simulink model "quadFly"  (R2019b)
settings: Solver=ode4  StartTime=0.0  StopTime=inf  FixedStep=0.001  RelTol=1e-3
InitFcn:
  | Init_control;
values from neighbouring files (symbols this model uses):
  Kd_RP_AgngleRate = 0.005    [Init_control.m]    (also in quadFly.sldd)
  Kd_YAW_AngleRate = 0.05    [Init_control.m]    (also in quadFly.sldd)
  Ki_RP_AgngleRate = 0.01    [Init_control.m]    (also in quadFly.sldd)
  Ki_YAW_AngleRate = 0.8    [Init_control.m]    (also in quadFly.sldd)
  Kp_RP_AgngleRate = 0.55    [Init_control.m]    (also in quadFly.sldd)
  Kp_RP_ANGLE = 6.5    [Init_control.m]    (also in quadFly.sldd)
  Kp_YAW_AngleRate = 3.2    [Init_control.m]    (also in quadFly.sldd)
  MAX_CONTROL_ANGLE_RATE_Y = 90    [Init_control.m]    (also in quadFly.sldd = 90.0)
  ModelInit_RPM = 0.0    [quadFly.sldd]
  ModelParam_envAltitude = -41.5260009765625    [quadFly.sldd]
  ModelParam_GlobalNoiseGainSwitch = 1.0    [quadFly.sldd]
  ModelParam_GPSLatLong = 40.1540302 116.2593683    [quadFly.sldd]
  ModelParam_motorCr = 1148.0    [quadFly.sldd]
  ModelParam_motorJm = 0.0001287    [quadFly.sldd]
  ModelParam_motorMinThr = 0.05    [quadFly.sldd]
  ModelParam_motorT = 0.02    [quadFly.sldd]
  ModelParam_motorWb = -141.4    [quadFly.sldd]
  ModelParam_rotorCm = 1.779E-7    [quadFly.sldd]
  ModelParam_rotorCt = 1.105E-5    [quadFly.sldd]
  ModelParam_uavCCm = 0.01 0.01 0.0055    [quadFly.sldd]
  ModelParam_uavCd = 0.073    [quadFly.sldd]
  ModelParam_uavDearo = 0.12    [quadFly.sldd]
  ModelParam_uavJ = 0.0211 0.0 0.0 0.0 0.0219 0.0 0.0 0.0 0.0366    [quadFly.sldd]
  ModelParam_uavMass = 1.4    [quadFly.sldd]
  ModelParam_uavR = 0.225    [quadFly.sldd]
  ModelParam_uavType = 3    [quadFly.sldd]
undefined symbols (not defined in the file or in its folder): DWORK0, DWORK1, DWORK10, DWORK11, DWORK12, DWORK13, DWORK14, DWORK15, DWORK2, DWORK3, DWORK4, DWORK5, DWORK6, DWORK7, DWORK8, DWORK9, earthRadius, KiPitchAttitude, KiRollAttitude, Receive, Send
libraries: simulink x15, ctrl_ADRC_angular_rate x4, aerolibfltsims x3, ctrl_ADRC_TD x2, shared6dof x1, aerolibanimutils x1
(part 2 of 4)

== system quadFly/Quadcopter Dynamics/Fail Model ==
  6DOF Bus : Inport
  Fail Model_sfcn : S-Function  FunctionName=Fail_sf  Parameters=sfcnParam1, sfcnParam2, sfcnParam3  SFunctionModules=""  SFunctionDeploymentMode=off  EnableBusSupport=off  mask{rtw_sf_name=Fail_sf, showVar=off, sfcnParam1=sfcnParam1, sfcnParam2=sfcnParam2, sfcnParam3=sfcnParam3}
      mask prompts: rtw_sf_name "Simulink:masks:GenSFuncName_MP"; showVar "Simulink:masks:GenSFuncShowModuleList_MP"; sfcnParam1 "ModelParam_uavJ:"; sfcnParam2 "ModelParam_uavMass:"; sfcnParam3 "ModelParam_uavR:"
      mask help: Simulink:masks:GenSFuncDesc_MD
      mask init: same as quadFly/Quadcopter Dynamics/Battery Model/Battery Model_sfcn
      settings: CopyFcn=|
      | if ~strcmp(get_param(gcb,'Linkstatus'),'none') && ...
      | ~strcmp(get_param(gcb,'Linkstatus'),'implicit')
      |   set_param(gcb,'LinkStatus','none');
      | end
      mask Help: eval('feval(''rtwprivate'',''rtwhelpview'',''rtw_sfcn_block'')');
      mask Display:
      | port_label('input',1,'Ve');
      | port_label('input',2,'Xe');
      | port_label('input',3,'Eular(rad)');
      | port_label('input',4,'DCM');
      | port_label('input',5,'Vb');
      | port_label('input',6,'wb');
      | port_label('input',7,'dwb/dt');
      | port_label('output',1,'m');
      | port_label('output',2,'J');
      | port_label('output',3,'dM');
  __InputSSForSFun__ : Subsystem
  __OutputSSForSFun__ : Subsystem
  Fail Model Bus : Outport  VectorParamsAs1DForOutWhenUnconnected=off
  wires:
  6DOF Bus/1 -> __InputSSForSFun__/1(6DOF Bus)
  __InputSSForSFun__/1(__UniqueOutportName__1__) -> Fail Model_sfcn/1
  __InputSSForSFun__/2(__UniqueOutportName__2__) -> Fail Model_sfcn/2
  __InputSSForSFun__/3(__UniqueOutportName__3__) -> Fail Model_sfcn/3
  __InputSSForSFun__/4(__UniqueOutportName__4__) -> Fail Model_sfcn/4
  __InputSSForSFun__/5(__UniqueOutportName__5__) -> Fail Model_sfcn/5
  __InputSSForSFun__/6(__UniqueOutportName__6__) -> Fail Model_sfcn/6
  __InputSSForSFun__/7(__UniqueOutportName__7__) -> Fail Model_sfcn/7
  Fail Model_sfcn/1 -> __OutputSSForSFun__/1(__UniqueInportName__1__)
  Fail Model_sfcn/2 -> __OutputSSForSFun__/2(__UniqueInportName__2__)
  Fail Model_sfcn/3 -> __OutputSSForSFun__/3(__UniqueInportName__3__)
  __OutputSSForSFun__/1(Fail Model Bus) -> Fail Model Bus/1

== system quadFly/Quadcopter Dynamics/Force and Moment Model ==
  MotorRads : Inport
  Environment Model Bus : Inport  Port=2
  6DOF Bus : Inport  Port=3
  Fail Model Bus : Inport  Port=4
  "tZ " : Inport  Port=5
  Force and Moment Model_sfcn : S-Function  FunctionName=Force_sf  Parameters=sfcnParam1, sfcnParam2, sfcnParam3, sfcnParam4, sfcnParam5, sfcnParam6, sfcnParam7, sfcnParam8  SFunctionModules=""  SFunctionDeploymentMode=off  EnableBusSupport=off  mask{rtw_sf_name=Force_sf, showVar=off, sfcnParam1=sfcnParam1, sfcnParam2=sfcnParam2, sfcnParam3=sfcnParam3, sfcnParam4=sfcnParam4, sfcnParam5=sfcnParam5, sfcnParam6=sfcnParam6, sfcnParam7=sfcnParam7, sfcnParam8=sfcnParam8}
      mask prompts: rtw_sf_name "Simulink:masks:GenSFuncName_MP"; showVar "Simulink:masks:GenSFuncShowModuleList_MP"; sfcnParam1 "ModelParam_motorJm:"; sfcnParam2 "ModelParam_rotorCm:"; sfcnParam3 "ModelParam_rotorCt:"; sfcnParam4 "ModelParam_uavCCm:"; sfcnParam5 "ModelParam_uavCd:"; sfcnParam6 "ModelParam_uavDearo:"; sfcnParam7 "ModelParam_uavR:"; sfcnParam8 "ModelParam_uavType:"
      mask help: Simulink:masks:GenSFuncDesc_MD
      mask init: same as quadFly/Quadcopter Dynamics/Battery Model/Battery Model_sfcn
      settings: CopyFcn=|
      | if ~strcmp(get_param(gcb,'Linkstatus'),'none') && ...
      | ~strcmp(get_param(gcb,'Linkstatus'),'implicit')
      |   set_param(gcb,'LinkStatus','none');
      | end
      mask Help: eval('feval(''rtwprivate'',''rtwhelpview'',''rtw_sfcn_block'')');
      mask Display:
      | port_label('input',1,'MotorRads');
      | port_label('input',2,'PosGPS');
      | port_label('input',3,'gravity');
      | port_label('input',4,'TempC');
      | port_label('input',5,'AirPressure');
      | port_label('input',6,'Rho');
      | port_label('input',7,'Windb');
      | port_label('input',8,'Wind');
      | port_label('input',9,'Ve');
      | port_label('input',10,'Xe');
      | port_label('input',11,'Eular(rad)');
      | port_label('input',12,'DCM');
      | port_label('input',13,'Vb');
      | port_label('input',14,'wb');
      | port_label('input',15,'dwb/dt');
      | port_label('input',16,'m');
      | port_label('input',17,'J');
      | port_label('input',18,'dM');
      | port_label('input',19,'tZ ');
      | port_label('output',1,'Fb');
      | port_label('output',2,'Mb');
      | port_label('output',3,'landed');
  __InputSSForSFun__ : Subsystem
  __OutputSSForSFun__ : Subsystem
  Force and Moment Model Bus : Outport  VectorParamsAs1DForOutWhenUnconnected=off
  wires:
  MotorRads/1 -> __InputSSForSFun__/1(MotorRads)
  Environment Model Bus/1 -> __InputSSForSFun__/2(Environment Model Bus)
  6DOF Bus/1 -> __InputSSForSFun__/3(6DOF Bus)
  Fail Model Bus/1 -> __InputSSForSFun__/4(Fail Model Bus)
  "tZ "/1 -> __InputSSForSFun__/5("tZ ")
  __InputSSForSFun__/1(__UniqueOutportName__1__) -> Force and Moment Model_sfcn/1
  __InputSSForSFun__/2(__UniqueOutportName__2__) -> Force and Moment Model_sfcn/2
  __InputSSForSFun__/3(__UniqueOutportName__3__) -> Force and Moment Model_sfcn/3
  __InputSSForSFun__/4(__UniqueOutportName__4__) -> Force and Moment Model_sfcn/4
  __InputSSForSFun__/5(__UniqueOutportName__5__) -> Force and Moment Model_sfcn/5
  __InputSSForSFun__/6(__UniqueOutportName__6__) -> Force and Moment Model_sfcn/6
  __InputSSForSFun__/7(__UniqueOutportName__7__) -> Force and Moment Model_sfcn/7
  __InputSSForSFun__/8(__UniqueOutportName__8__) -> Force and Moment Model_sfcn/8
  __InputSSForSFun__/9(__UniqueOutportName__9__) -> Force and Moment Model_sfcn/9
  __InputSSForSFun__/10(__UniqueOutportName__10__) -> Force and Moment Model_sfcn/10
  __InputSSForSFun__/11(__UniqueOutportName__11__) -> Force and Moment Model_sfcn/11
  __InputSSForSFun__/12(__UniqueOutportName__12__) -> Force and Moment Model_sfcn/12
  __InputSSForSFun__/13(__UniqueOutportName__13__) -> Force and Moment Model_sfcn/13
  __InputSSForSFun__/14(__UniqueOutportName__14__) -> Force and Moment Model_sfcn/14
  __InputSSForSFun__/15(__UniqueOutportName__15__) -> Force and Moment Model_sfcn/15
  __InputSSForSFun__/16(__UniqueOutportName__16__) -> Force and Moment Model_sfcn/16
  __InputSSForSFun__/17(__UniqueOutportName__17__) -> Force and Moment Model_sfcn/17
  __InputSSForSFun__/18(__UniqueOutportName__18__) -> Force and Moment Model_sfcn/18
  __InputSSForSFun__/19(__UniqueOutportName__19__) -> Force and Moment Model_sfcn/19
  Force and Moment Model_sfcn/1 -> __OutputSSForSFun__/1(__UniqueInportName__1__)
  Force and Moment Model_sfcn/2 -> __OutputSSForSFun__/2(__UniqueInportName__2__)
  Force and Moment Model_sfcn/3 -> __OutputSSForSFun__/3(__UniqueInportName__3__)
  __OutputSSForSFun__/1(Force and Moment Model Bus) -> Force and Moment Model Bus/1

== system quadFly/Quadcopter Dynamics/Motor Model ==
  Battery Model Bus : Inport
  Motor Model_sfcn : S-Function  FunctionName=Motor_sf  Parameters=sfcnParam1, sfcnParam2, sfcnParam3, sfcnParam4, sfcnParam5  SFunctionModules=""  SFunctionDeploymentMode=off  EnableBusSupport=off  mask{rtw_sf_name=Motor_sf, showVar=off, sfcnParam1=sfcnParam1, sfcnParam2=sfcnParam2, sfcnParam3=sfcnParam3, sfcnParam4=sfcnParam4, sfcnParam5=sfcnParam5}
      mask prompts: rtw_sf_name "Simulink:masks:GenSFuncName_MP"; showVar "Simulink:masks:GenSFuncShowModuleList_MP"; sfcnParam1 "ModelInit_RPM:"; sfcnParam2 "ModelParam_motorCr:"; sfcnParam3 "ModelParam_motorMinThr:"; sfcnParam4 "ModelParam_motorT:"; sfcnParam5 "ModelParam_motorWb:"
      mask help: Simulink:masks:GenSFuncDesc_MD
      mask init: same as quadFly/Quadcopter Dynamics/Battery Model/Battery Model_sfcn
      settings: CopyFcn=|
      | if ~strcmp(get_param(gcb,'Linkstatus'),'none') && ...
      | ~strcmp(get_param(gcb,'Linkstatus'),'implicit')
      |   set_param(gcb,'LinkStatus','none');
      | end
      mask Help: eval('feval(''rtwprivate'',''rtwhelpview'',''rtw_sfcn_block'')');
      mask Display:
      | port_label('input',1,'PWMOut');
      | port_label('input',2,'cellVol');
      | port_label('input',3,'remCapa');
      | port_label('output',1,'MotorRads');
  __InputSSForSFun__ : Subsystem
  __OutputSSForSFun__ : Subsystem
  MotorRads : Outport  VectorParamsAs1DForOutWhenUnconnected=off
  wires:
  Battery Model Bus/1 -> __InputSSForSFun__/1(Battery Model Bus)
  __InputSSForSFun__/1(__UniqueOutportName__1__) -> Motor Model_sfcn/1
  __InputSSForSFun__/2(__UniqueOutportName__2__) -> Motor Model_sfcn/2
  __InputSSForSFun__/3(__UniqueOutportName__3__) -> Motor Model_sfcn/3
  Motor Model_sfcn/1 -> __OutputSSForSFun__/1(__UniqueInportName__1__)
  __OutputSSForSFun__/1(MotorRads) -> MotorRads/1

== system quadFly/Quadcopter Dynamics/OutputPort ==
  Environment Model Bus : Inport
  MotorRads : Inport  Port=2
  zt : Inport  Port=3
  Force and Moment Model Bus : Inport  Port=4
  6DOF Bus : Inport  Port=5
  Fail Model Bus : Inport  Port=6
  Battery Model Bus : Inport  Port=7
  OutputPort_sfcn : S-Function  FunctionName=OutputPort_sf  Parameters=sfcnParam1, sfcnParam2, sfcnParam3  SFunctionModules=""  SFunctionDeploymentMode=off  EnableBusSupport=off  SFcnStateName=DWORK0,DWORK1,DWORK2,DWORK3,DWORK4,DWORK5,DWORK6,DWORK7,DWORK8,DWORK9  mask{rtw_sf_name=OutputPort_sf, showVar=off, sfcnParam1=sfcnParam1, sfcnParam2=sfcnParam2, sfcnParam3=sfcnParam3}
      mask prompts: rtw_sf_name "Simulink:masks:GenSFuncName_MP"; showVar "Simulink:masks:GenSFuncShowModuleList_MP"; sfcnParam1 "ModelParam_GPSLatLong:"; sfcnParam2 "ModelParam_GlobalNoiseGainSwitch:"; sfcnParam3 "ModelParam_envAltitude:"
      mask help: Simulink:masks:GenSFuncDesc_MD
      mask init: same as quadFly/Quadcopter Dynamics/Battery Model/Battery Model_sfcn
      settings: SFcnIsStateOwnerBlock=on
      settings: CopyFcn=|
      | if ~strcmp(get_param(gcb,'Linkstatus'),'none') && ...
      | ~strcmp(get_param(gcb,'Linkstatus'),'implicit')
      |   set_param(gcb,'LinkStatus','none');
      | end
      mask Help: eval('feval(''rtwprivate'',''rtwhelpview'',''rtw_sfcn_block'')');
      mask Display:
      | port_label('input',1,'PosGPS');
      | port_label('input',2,'gravity');
      | port_label('input',3,'TempC');
      | port_label('input',4,'AirPressure');
      | port_label('input',5,'Rho');
      | port_label('input',6,'Windb');
      | port_label('input',7,'Wind');
      | port_label('input',8,'MotorRads');
      | port_label('input',9,'zt');
      | port_label('input',10,'Fb');
      | port_label('input',11,'Mb');
      | port_label('input',12,'landed');
      | port_label('input',13,'Ve');
      | port_label('input',14,'Xe');
      | port_label('input',15,'Eular(rad)');
      | port_label('input',16,'DCM');
      | port_label('input',17,'Vb');
      | port_label('input',18,'wb');
      | port_label('input',19,'dwb/dt');
      | port_label('input',20,'m');
      | port_label('input',21,'J');
      | port_label('input',22,'dM');
      | port_label('input',23,'PWMOut');
      | port_label('input',24,'cellVol');
      | port_label('input',25,'remCapa');
      | port_label('output',1,'MavLinkSensorData');
      | port_label('output',2,'MavLinkStateQuatData');
      | port_label('output',3,'MavLinkGPSData');
      | port_label('output',4,'HILGPS');
      | port_label('output',5,'MagDec');
      | port_label('output',6,'SysTime');
      | port_label('output',7,'VelE');
      | port_label('output',8,'PosE');
      | port_label('output',9,'AngEuler');
      | port_label('output',10,'AngQuatern');
      | port_label('output',11,'PosGPSb');
      | port_label('output',12,'RateB');
      | port_label('output',13,'AccB');
      | port_label('output',14,'FailInfo');
      | port_label('output',15,'landedb');
      | port_label('output',16,'BattCellVoltage');
      | port_label('output',17,'BattRemCapacity');
      | port_label('output',18,'MotorRPMS');
      | port_label('output',19,'wind');
  __InputSSForSFun__ : Subsystem
  __OutputSSForSFun__ : Subsystem
  MavLinkSensorData : Outport  OutDataTypeStr=Bus: MavLinkSensor  SampleTime=[-1 0]  VectorParamsAs1DForOutWhenUnconnected=off  BusOutputAsStruct=on
  MavLinkStateQuatData : Outport  Port=2  OutDataTypeStr=Bus: MavLinkStateQuat  SampleTime=[-1 0]  VectorParamsAs1DForOutWhenUnconnected=off  BusOutputAsStruct=on
  MavLinkGPSData : Outport  Port=3  OutDataTypeStr=Bus: MavLinkGPS  SampleTime=[-1 0]  VectorParamsAs1DForOutWhenUnconnected=off  BusOutputAsStruct=on
  HILGPS : Outport  Port=4  OutDataTypeStr=Bus: HILGPS  SampleTime=[-1 0]  VectorParamsAs1DForOutWhenUnconnected=off  BusOutputAsStruct=on
  MagDec : Outport  Port=5  VectorParamsAs1DForOutWhenUnconnected=off
  SysTime : Outport  Port=6  VectorParamsAs1DForOutWhenUnconnected=off
  VelE : Outport  Port=7  VectorParamsAs1DForOutWhenUnconnected=off
  PosE : Outport  Port=8  VectorParamsAs1DForOutWhenUnconnected=off
  AngEuler : Outport  Port=9  VectorParamsAs1DForOutWhenUnconnected=off
  AngQuatern : Outport  Port=10  VectorParamsAs1DForOutWhenUnconnected=off
  PosGPS : Outport  Port=11  VectorParamsAs1DForOutWhenUnconnected=off
  RateB : Outport  Port=12  VectorParamsAs1DForOutWhenUnconnected=off
  AccB : Outport  Port=13  VectorParamsAs1DForOutWhenUnconnected=off
  FailInfo : Outport  Port=14  VectorParamsAs1DForOutWhenUnconnected=off
  landed : Outport  Port=15  VectorParamsAs1DForOutWhenUnconnected=off
  BattCellVoltage : Outport  Port=16  VectorParamsAs1DForOutWhenUnconnected=off
  BattRemCapacity : Outport  Port=17  VectorParamsAs1DForOutWhenUnconnected=off
  MotorRPMS : Outport  Port=18  VectorParamsAs1DForOutWhenUnconnected=off
  wind : Outport  Port=19  VectorParamsAs1DForOutWhenUnconnected=off
  wires:
  Environment Model Bus/1 -> __InputSSForSFun__/1(Environment Model Bus)
  MotorRads/1 -> __InputSSForSFun__/2(MotorRads)
  zt/1 -> __InputSSForSFun__/3(zt)
  Force and Moment Model Bus/1 -> __InputSSForSFun__/4(Force and Moment Model Bus)
  6DOF Bus/1 -> __InputSSForSFun__/5(6DOF Bus)
  Fail Model Bus/1 -> __InputSSForSFun__/6(Fail Model Bus)
  Battery Model Bus/1 -> __InputSSForSFun__/7(Battery Model Bus)
  __InputSSForSFun__/1(__UniqueOutportName__1__) -> OutputPort_sfcn/1
  __InputSSForSFun__/2(__UniqueOutportName__2__) -> OutputPort_sfcn/2
  __InputSSForSFun__/3(__UniqueOutportName__3__) -> OutputPort_sfcn/3
  __InputSSForSFun__/4(__UniqueOutportName__4__) -> OutputPort_sfcn/4
  __InputSSForSFun__/5(__UniqueOutportName__5__) -> OutputPort_sfcn/5
  __InputSSForSFun__/6(__UniqueOutportName__6__) -> OutputPort_sfcn/6
  __InputSSForSFun__/7(__UniqueOutportName__7__) -> OutputPort_sfcn/7
  __InputSSForSFun__/8(__UniqueOutportName__8__) -> OutputPort_sfcn/8
  __InputSSForSFun__/9(__UniqueOutportName__9__) -> OutputPort_sfcn/9
  __InputSSForSFun__/10(__UniqueOutportName__10__) -> OutputPort_sfcn/10
  __InputSSForSFun__/11(__UniqueOutportName__11__) -> OutputPort_sfcn/11
  __InputSSForSFun__/12(__UniqueOutportName__12__) -> OutputPort_sfcn/12
  __InputSSForSFun__/13(__UniqueOutportName__13__) -> OutputPort_sfcn/13
  __InputSSForSFun__/14(__UniqueOutportName__14__) -> OutputPort_sfcn/14
  __InputSSForSFun__/15(__UniqueOutportName__15__) -> OutputPort_sfcn/15
  __InputSSForSFun__/16(__UniqueOutportName__16__) -> OutputPort_sfcn/16
  __InputSSForSFun__/17(__UniqueOutportName__17__) -> OutputPort_sfcn/17
  __InputSSForSFun__/18(__UniqueOutportName__18__) -> OutputPort_sfcn/18
  __InputSSForSFun__/19(__UniqueOutportName__19__) -> OutputPort_sfcn/19
  __InputSSForSFun__/20(__UniqueOutportName__20__) -> OutputPort_sfcn/20
  __InputSSForSFun__/21(__UniqueOutportName__21__) -> OutputPort_sfcn/21
  __InputSSForSFun__/22(__UniqueOutportName__22__) -> OutputPort_sfcn/22
  __InputSSForSFun__/23(__UniqueOutportName__23__) -> OutputPort_sfcn/23
  __InputSSForSFun__/24(__UniqueOutportName__24__) -> OutputPort_sfcn/24
  __InputSSForSFun__/25(__UniqueOutportName__25__) -> OutputPort_sfcn/25
  OutputPort_sfcn/1 -> __OutputSSForSFun__/1(__UniqueInportName__1__)
  OutputPort_sfcn/2 -> __OutputSSForSFun__/2(__UniqueInportName__2__)
  OutputPort_sfcn/3 -> __OutputSSForSFun__/3(__UniqueInportName__3__)
  OutputPort_sfcn/4 -> __OutputSSForSFun__/4(__UniqueInportName__4__)
  OutputPort_sfcn/5 -> __OutputSSForSFun__/5(__UniqueInportName__5__)
  OutputPort_sfcn/6 -> __OutputSSForSFun__/6(__UniqueInportName__6__)
  OutputPort_sfcn/7 -> __OutputSSForSFun__/7(__UniqueInportName__7__)
  OutputPort_sfcn/8 -> __OutputSSForSFun__/8(__UniqueInportName__8__)
  OutputPort_sfcn/9 -> __OutputSSForSFun__/9(__UniqueInportName__9__)
  OutputPort_sfcn/10 -> __OutputSSForSFun__/10(__UniqueInportName__10__)
  OutputPort_sfcn/11 -> __OutputSSForSFun__/11(__UniqueInportName__11__)
  OutputPort_sfcn/12 -> __OutputSSForSFun__/12(__UniqueInportName__12__)
  OutputPort_sfcn/13 -> __OutputSSForSFun__/13(__UniqueInportName__13__)
  OutputPort_sfcn/14 -> __OutputSSForSFun__/14(__UniqueInportName__14__)
  OutputPort_sfcn/15 -> __OutputSSForSFun__/15(__UniqueInportName__15__)
  OutputPort_sfcn/16 -> __OutputSSForSFun__/16(__UniqueInportName__16__)
  OutputPort_sfcn/17 -> __OutputSSForSFun__/17(__UniqueInportName__17__)
  OutputPort_sfcn/18 -> __OutputSSForSFun__/18(__UniqueInportName__18__)
  OutputPort_sfcn/19 -> __OutputSSForSFun__/19(__UniqueInportName__19__)
  __OutputSSForSFun__/1(MavLinkSensorData) -> MavLinkSensorData/1
  __OutputSSForSFun__/2(MavLinkStateQuatData) -> MavLinkStateQuatData/1
  __OutputSSForSFun__/3(MavLinkGPSData) -> MavLinkGPSData/1
  __OutputSSForSFun__/4(HILGPS) -> HILGPS/1
  __OutputSSForSFun__/5(MagDec) -> MagDec/1
  __OutputSSForSFun__/6(SysTime) -> SysTime/1
  __OutputSSForSFun__/7(VelE) -> VelE/1
  __OutputSSForSFun__/8(PosE) -> PosE/1
  __OutputSSForSFun__/9(AngEuler) -> AngEuler/1
  __OutputSSForSFun__/10(AngQuatern) -> AngQuatern/1
  __OutputSSForSFun__/11(PosGPS) -> PosGPS/1
  __OutputSSForSFun__/12(RateB) -> RateB/1
  __OutputSSForSFun__/13(AccB) -> AccB/1
  __OutputSSForSFun__/14(FailInfo) -> FailInfo/1
  __OutputSSForSFun__/15(landed) -> landed/1
  __OutputSSForSFun__/16(BattCellVoltage) -> BattCellVoltage/1
  __OutputSSForSFun__/17(BattRemCapacity) -> BattRemCapacity/1
  __OutputSSForSFun__/18(MotorRPMS) -> MotorRPMS/1
  __OutputSSForSFun__/19(wind) -> wind/1

== system quadFly/Quadcopter Dynamics/Separation of float Data1 ==
  note: 小数部分
  float_Data : Inport
  Add2 : Sum  Inputs=+-
  Integer Uint : Constant  Value=IntUint
  Math Function1 : Math  Operator=mod  SaturateOnIntegerOverflow=on
  Integer_Part : Outport  VectorParamsAs1DForOutWhenUnconnected=off
  decimalt_Part : Outport  Port=2  VectorParamsAs1DForOutWhenUnconnected=off
  wires:
  Math Function1/1 -> decimalt_Part/1, Add2/2
  Integer Uint/1 -> Math Function1/2
  Add2/1 -> Integer_Part/1
  float_Data/1 -> Math Function1/1, Add2/1

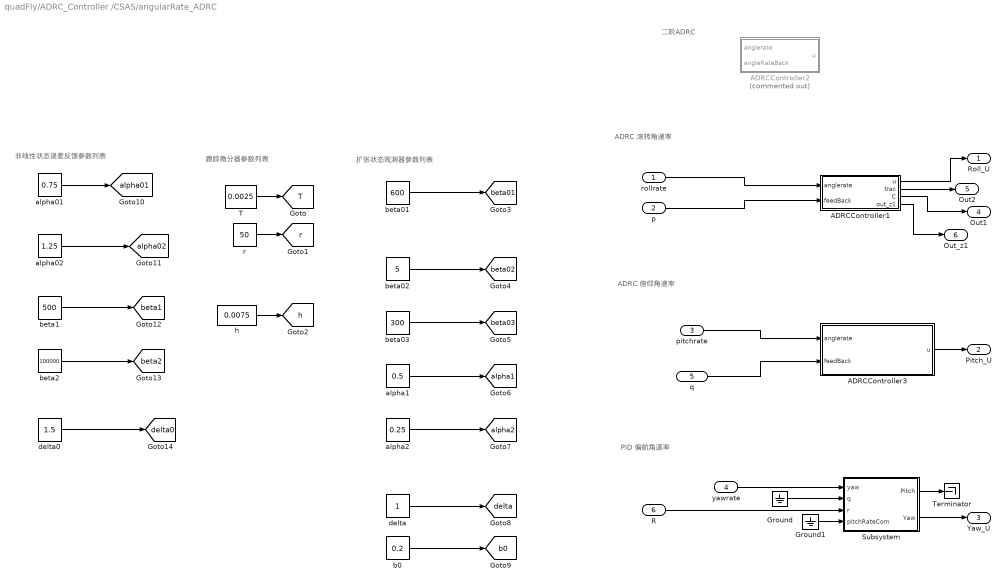
== system quadFly/ADRC_Controller /CSAS/angularRate_ADRC ==
  note: ADRC 俯仰角速率
  note: 二阶ADRC
  note: PID 偏航角速率
  note: ADRC 滚转角速率
  note: 非线性状态误差反馈参数列表
  note: 扩张状态观测器参数列表
  note: 跟踪微分器参数列表
  rollrate : Inport
  p : Inport  Port=2
  pitchrate : Inport  Port=3
  yawrate : Inport  Port=4
  q : Inport  Port=5
  R : Inport  Port=6
  ADRCController1 : Subsystem
  ADRCController2 : Subsystem  Commented=on
  ADRCController3 : Subsystem
  Ground : Ground
  Ground1 : Ground
  Subsystem : Subsystem
  T : Constant  Value=0.0025
  Terminator : Terminator
  alpha01 : Constant  Value=0.75
  alpha02 : Constant  Value=1.25
  alpha1 : Constant  Value=0.5
  alpha2 : Constant  Value=0.25
  b0 : Constant  Value=0.2
  beta01 : Constant  Value=600
  beta02 : Constant  Value=5
  beta03 : Constant  Value=300
  beta1 : Constant  Value=500
  beta2 : Constant  Value=100000
  delta : Constant
  delta0 : Constant  Value=1.5
  h : Constant  Value=0.0075
  r : Constant  Value=50
  Roll_U : Outport
  Pitch_U : Outport  Port=2
  Yaw_U : Outport  Port=3
  Out1 : Outport  Port=4
  Out2 : Outport  Port=5
  Out_z1 : Outport  Port=6
  tag scope: T=global, alpha01=global, alpha02=global, alpha1=global, alpha2=global, b0=global, beta01=global, beta02=global, beta03=global, beta1=global, beta2=global, delta0=global, delta=global, h=global, r=global
  wires:
  ADRCController1/1(u) -> Roll_U/1
  rollrate/1 -> ADRCController1/1(anglerate)
  T/1 -> [T]
  beta02/1 -> [beta02]
  r/1 -> [r]
  h/1 -> [h]
  beta01/1 -> [beta01]
  alpha1/1 -> [alpha1]
  beta03/1 -> [beta03]
  alpha2/1 -> [alpha2]
  delta/1 -> [delta]
  b0/1 -> [b0]
  alpha01/1 -> [alpha01]
  alpha02/1 -> [alpha02]
  beta1/1 -> [beta1]
  beta2/1 -> [beta2]
  delta0/1 -> [delta0]
  p/1 -> ADRCController1/2(feedBack)
  yawrate/1 -> Subsystem/1(yaw)
  Subsystem/2(Yaw) -> Yaw_U/1
  pitchrate/1 -> ADRCController3/1(anglerate)
  R/1 -> Subsystem/3(r)
  Subsystem/1(Pitch) -> Terminator/1
  q/1 -> ADRCController3/2(feedBack)
  ADRCController1/3(C) -> Out1/1
  ADRCController1/2(trac) -> Out2/1
  ADRCController1/4(out_z1) -> Out_z1/1
  Ground1/1 -> Subsystem/4(pitchRateCom)
  Ground/1 -> Subsystem/2(q)
  ADRCController3/1(u) -> Pitch_U/1

== system quadFly/ADRC_Controller /CSAS/angular_PID ==
  Roll : Inport
  Pitch : Inport  Port=2
  phi : Inport  Port=3
  theta : Inport  Port=4
  posai : Inport  Port=5
  yaw : Inport  Port=6
  Sum : Sum  Inputs=|+-
  Sum1 : Sum  Inputs=|+-
  Sum2 : Sum  Inputs=|+-
  pitch_attitude1 : simulink/Continuous/PID Controller  Controller=P  Form=Parallel  TimeDomain=Discrete-time  SampleTime=-1  IntegratorMethod=Forward Euler  FilterMethod=Forward Euler  ControllerParametersSource=internal  P=Kp_RP_ANGLE  I=KiRollAttitude  D=0.01  UseFilter=on  N=100  TunerSelectOption=Transfer Function Based (PID Tuner App)  InitialConditionSource=internal  InitialConditionForIntegrator=0  InitialConditionForFilter=0  DifferentiatorICPrevScaledInput=0  ExternalReset=none  TrackingMode=off  Kt=1  LimitOutput=on  UpperSaturationLimit=180  LowerSaturationLimit=-180  LinearizeAsGain=on  AntiWindupMode=back-calculation  Kb=1  POutMin=[]  POutMax=[]  IOutMin=[]  IOutMax=[]  DOutMin=[]  DOutMax=[]  NOutMin=[]  NOutMax=[]  SumOutMin=[]  SumOutMax=[]  SaturationOutMin=[]  SaturationOutMax=[]  PParamMin=[]  PParamMax=[]  IParamMin=[]  IParamMax=[]  DParamMin=[]  DParamMax=[]  NParamMin=[]  NParamMax=[]  KbParamMin=[]  KbParamMax=[]  KtParamMin=[]  KtParamMax=[]  KbOutMin=[]  KbOutMax=[]  KtOutMin=[]  KtOutMax=[]  IntegratorOutMin=[]  IntegratorOutMax=[]  FilterOutMin=[]  FilterOutMax=[]  SumI1OutMin=[]  SumI1OutMax=[]  SumI2OutMin=[]  SumI2OutMax=[]  SumI3OutMin=[]  SumI3OutMax=[]  SumI4OutMin=[]  SumI4OutMax=[]  SumDOutMin=[]  SumDOutMax=[]  DifferentiatorOutMin=[]  DifferentiatorOutMax=[]  FilterDiffOutCoefMin=[]  FilterDiffOutCoefMax=[]  ReciprocalOutMin=[]  ReciprocalOutMax=[]  SumDenOutMin=[]  SumDenOutMax=[]  SumNumOutMin=[]  SumNumOutMax=[]  DivideOutMin=[]  DivideOutMax=[]  IntegratorContinuousStateAttributes=''  IntegratorStateMustResolveToSignalObject=off  IntegratorRTWStateStorageClass=Auto  FilterContinuousStateAttributes=''  FilterStateMustResolveToSignalObject=off  FilterRTWStateStorageClass=Auto  ParallelPVariant=InternalParameters  IdealPVariant=Disabled  IVariant=Disabled  DVariant=Disabled  IntegratorVariant=Disabled  SatVariant=Enabled  AWVariant=Disabled  PCopyVariant=Disabled  TRVariant=Disabled  FdbkBlocksVariant=Forward  IdealPFdbkVariant=Disabled  SatFdbkVariant=Disabled  DerivativeFilterVariant=Disabled  NVariant=Disabled  NCopyVariant=Disabled_SignalSpec  FilterICVariant=Disabled  IntegratorICVariant=Disabled  ExternalResetVariant=Disabled  TRSumVariant=Passthrough  SumFdbkVariant=Disabled  SumVariant=Passthrough_P
  roll_attitude : simulink/Continuous/PID Controller  Controller=P  Form=Parallel  TimeDomain=Discrete-time  SampleTime=-1  IntegratorMethod=Forward Euler  FilterMethod=Forward Euler  ControllerParametersSource=internal  P=3.5  I=0.002  D=0.01  UseFilter=on  N=100  TunerSelectOption=Transfer Function Based (PID Tuner App)  InitialConditionSource=internal  InitialConditionForIntegrator=0  InitialConditionForFilter=0  DifferentiatorICPrevScaledInput=0  ExternalReset=none  TrackingMode=off  Kt=1  LimitOutput=on  UpperSaturationLimit=180  LowerSaturationLimit=-180  LinearizeAsGain=on  AntiWindupMode=back-calculation  Kb=1  POutMin=[]  POutMax=[]  IOutMin=[]  IOutMax=[]  DOutMin=[]  DOutMax=[]  NOutMin=[]  NOutMax=[]  SumOutMin=[]  SumOutMax=[]  SaturationOutMin=[]  SaturationOutMax=[]  PParamMin=[]  PParamMax=[]  IParamMin=[]  IParamMax=[]  DParamMin=[]  DParamMax=[]  NParamMin=[]  NParamMax=[]  KbParamMin=[]  KbParamMax=[]  KtParamMin=[]  KtParamMax=[]  KbOutMin=[]  KbOutMax=[]  KtOutMin=[]  KtOutMax=[]  IntegratorOutMin=[]  IntegratorOutMax=[]  FilterOutMin=[]  FilterOutMax=[]  SumI1OutMin=[]  SumI1OutMax=[]  SumI2OutMin=[]  SumI2OutMax=[]  SumI3OutMin=[]  SumI3OutMax=[]  SumI4OutMin=[]  SumI4OutMax=[]  SumDOutMin=[]  SumDOutMax=[]  DifferentiatorOutMin=[]  DifferentiatorOutMax=[]  FilterDiffOutCoefMin=[]  FilterDiffOutCoefMax=[]  ReciprocalOutMin=[]  ReciprocalOutMax=[]  SumDenOutMin=[]  SumDenOutMax=[]  SumNumOutMin=[]  SumNumOutMax=[]  DivideOutMin=[]  DivideOutMax=[]  IntegratorContinuousStateAttributes=''  IntegratorStateMustResolveToSignalObject=off  IntegratorRTWStateStorageClass=Auto  FilterContinuousStateAttributes=''  FilterStateMustResolveToSignalObject=off  FilterRTWStateStorageClass=Auto  ParallelPVariant=InternalParameters  IdealPVariant=Disabled  IVariant=Disabled  DVariant=Disabled  IntegratorVariant=Disabled  SatVariant=Enabled  AWVariant=Disabled  PCopyVariant=Disabled  TRVariant=Disabled  FdbkBlocksVariant=Forward  IdealPFdbkVariant=Disabled  SatFdbkVariant=Disabled  DerivativeFilterVariant=Disabled  NVariant=Disabled  NCopyVariant=Disabled_SignalSpec  FilterICVariant=Disabled  IntegratorICVariant=Disabled  ExternalResetVariant=Disabled  TRSumVariant=Passthrough  SumFdbkVariant=Disabled  SumVariant=Passthrough_P
  yaw_attitude2 : simulink/Continuous/PID Controller  Controller=P  Form=Parallel  TimeDomain=Discrete-time  SampleTime=-1  IntegratorMethod=Forward Euler  FilterMethod=Forward Euler  ControllerParametersSource=internal  P=Kp_RP_ANGLE  I=KiRollAttitude  D=0.01  UseFilter=on  N=100  TunerSelectOption=Transfer Function Based (PID Tuner App)  InitialConditionSource=internal  InitialConditionForIntegrator=0  InitialConditionForFilter=0  DifferentiatorICPrevScaledInput=0  ExternalReset=none  TrackingMode=off  Kt=1  LimitOutput=on  UpperSaturationLimit=180  LowerSaturationLimit=-180  LinearizeAsGain=on  AntiWindupMode=back-calculation  Kb=1  POutMin=[]  POutMax=[]  IOutMin=[]  IOutMax=[]  DOutMin=[]  DOutMax=[]  NOutMin=[]  NOutMax=[]  SumOutMin=[]  SumOutMax=[]  SaturationOutMin=[]  SaturationOutMax=[]  PParamMin=[]  PParamMax=[]  IParamMin=[]  IParamMax=[]  DParamMin=[]  DParamMax=[]  NParamMin=[]  NParamMax=[]  KbParamMin=[]  KbParamMax=[]  KtParamMin=[]  KtParamMax=[]  KbOutMin=[]  KbOutMax=[]  KtOutMin=[]  KtOutMax=[]  IntegratorOutMin=[]  IntegratorOutMax=[]  FilterOutMin=[]  FilterOutMax=[]  SumI1OutMin=[]  SumI1OutMax=[]  SumI2OutMin=[]  SumI2OutMax=[]  SumI3OutMin=[]  SumI3OutMax=[]  SumI4OutMin=[]  SumI4OutMax=[]  SumDOutMin=[]  SumDOutMax=[]  DifferentiatorOutMin=[]  DifferentiatorOutMax=[]  FilterDiffOutCoefMin=[]  FilterDiffOutCoefMax=[]  ReciprocalOutMin=[]  ReciprocalOutMax=[]  SumDenOutMin=[]  SumDenOutMax=[]  SumNumOutMin=[]  SumNumOutMax=[]  DivideOutMin=[]  DivideOutMax=[]  IntegratorContinuousStateAttributes=''  IntegratorStateMustResolveToSignalObject=off  IntegratorRTWStateStorageClass=Auto  FilterContinuousStateAttributes=''  FilterStateMustResolveToSignalObject=off  FilterRTWStateStorageClass=Auto  ParallelPVariant=InternalParameters  IdealPVariant=Disabled  IVariant=Disabled  DVariant=Disabled  IntegratorVariant=Disabled  SatVariant=Enabled  AWVariant=Disabled  PCopyVariant=Disabled  TRVariant=Disabled  FdbkBlocksVariant=Forward  IdealPFdbkVariant=Disabled  SatFdbkVariant=Disabled  DerivativeFilterVariant=Disabled  NVariant=Disabled  NCopyVariant=Disabled_SignalSpec  FilterICVariant=Disabled  IntegratorICVariant=Disabled  ExternalResetVariant=Disabled  TRSumVariant=Passthrough  SumFdbkVariant=Disabled  SumVariant=Passthrough_P
  roll_rate : Outport
  pitch_rate : Outport  Port=2
  yaw_rate : Outport  Port=3
  wires:
  Roll/1 -> Sum/1
  phi/1 -> Sum/2
  Sum/1 -> roll_attitude/1
  theta/1 -> Sum1/2
  Pitch/1 -> Sum1/1
  Sum1/1 -> pitch_attitude1/1
  yaw/1 -> Sum2/1
  posai/1 -> Sum2/2
  Sum2/1 -> yaw_attitude2/1
  roll_attitude/1 -> roll_rate/1
  pitch_attitude1/1 -> pitch_rate/1
  yaw_attitude2/1 -> yaw_rate/1

== system quadFly/Quadcopter Dynamics/Battery Model/__InputSSForSFun__ ==
  PWMin : Inport
  __UniqueOutportName__1__ : Outport  VectorParamsAs1DForOutWhenUnconnected=off
  wires:
  PWMin/1 -> __UniqueOutportName__1__/1

== system quadFly/Quadcopter Dynamics/Battery Model/__OutputSSForSFun__ ==
  __UniqueInportName__1__ : Inport
  __UniqueInportName__2__ : Inport  Port=2
  __UniqueInportName__3__ : Inport  Port=3
  Mux1 : BusCreator  Inputs=3
  Battery Model Bus : Outport  VectorParamsAs1DForOutWhenUnconnected=off
  wires:
  __UniqueInportName__1__/1 -> Mux1/1  "PWMOut"
  __UniqueInportName__2__/1 -> Mux1/2  "cellVol"
  __UniqueInportName__3__/1 -> Mux1/3  "remCapa"
  Mux1/1 -> Battery Model Bus/1

== system quadFly/Quadcopter Dynamics/Environment Model/__InputSSForSFun__ ==
  6DOF Bus : Inport
  temporaryBusSelectName_1 : BusSelector  OutputSignals=Ve,Xe,Eular(rad),DCM,Vb,wb,dwb/dt
  __UniqueOutportName__1__ : Outport  VectorParamsAs1DForOutWhenUnconnected=off
  __UniqueOutportName__2__ : Outport  Port=2  VectorParamsAs1DForOutWhenUnconnected=off
  __UniqueOutportName__3__ : Outport  Port=3  VectorParamsAs1DForOutWhenUnconnected=off
  __UniqueOutportName__4__ : Outport  Port=4  VectorParamsAs1DForOutWhenUnconnected=off
  __UniqueOutportName__5__ : Outport  Port=5  VectorParamsAs1DForOutWhenUnconnected=off
  __UniqueOutportName__6__ : Outport  Port=6  VectorParamsAs1DForOutWhenUnconnected=off
  __UniqueOutportName__7__ : Outport  Port=7  VectorParamsAs1DForOutWhenUnconnected=off
  wires:
  6DOF Bus/1 -> temporaryBusSelectName_1/1
  temporaryBusSelectName_1/1 -> __UniqueOutportName__1__/1  "<Ve>"
  temporaryBusSelectName_1/2 -> __UniqueOutportName__2__/1  "<Xe>"
  temporaryBusSelectName_1/3 -> __UniqueOutportName__3__/1  "<Eular(rad)>"
  temporaryBusSelectName_1/4 -> __UniqueOutportName__4__/1  "<DCM>"
  temporaryBusSelectName_1/5 -> __UniqueOutportName__5__/1  "<Vb>"
  temporaryBusSelectName_1/6 -> __UniqueOutportName__6__/1  "<wb>"
  temporaryBusSelectName_1/7 -> __UniqueOutportName__7__/1  "<dwb/dt>"

== system quadFly/Quadcopter Dynamics/Environment Model/__OutputSSForSFun__ ==
  __UniqueInportName__1__ : Inport
  __UniqueInportName__2__ : Inport  Port=2
  __UniqueInportName__3__ : Inport  Port=3
  __UniqueInportName__4__ : Inport  Port=4
  __UniqueInportName__5__ : Inport  Port=5
  __UniqueInportName__6__ : Inport  Port=6
  __UniqueInportName__7__ : Inport  Port=7
  Mux1 : BusCreator  Inputs=7
  Environment Model Bus : Outport  VectorParamsAs1DForOutWhenUnconnected=off
  wires:
  __UniqueInportName__1__/1 -> Mux1/1  "PosGPS"
  __UniqueInportName__2__/1 -> Mux1/2  "gravity"
  __UniqueInportName__3__/1 -> Mux1/3  "TempC"
  __UniqueInportName__4__/1 -> Mux1/4  "AirPressure"
  __UniqueInportName__5__/1 -> Mux1/5  "Rho"
  __UniqueInportName__6__/1 -> Mux1/6  "Windb"
  __UniqueInportName__7__/1 -> Mux1/7  "Wind"
  Mux1/1 -> Environment Model Bus/1

== system quadFly/Quadcopter Dynamics/Fail Model/__InputSSForSFun__ ==
  6DOF Bus : Inport
  temporaryBusSelectName_1 : BusSelector  OutputSignals=Ve,Xe,Eular(rad),DCM,Vb,wb,dwb/dt
  __UniqueOutportName__1__ : Outport  VectorParamsAs1DForOutWhenUnconnected=off
  __UniqueOutportName__2__ : Outport  Port=2  VectorParamsAs1DForOutWhenUnconnected=off
  __UniqueOutportName__3__ : Outport  Port=3  VectorParamsAs1DForOutWhenUnconnected=off
  __UniqueOutportName__4__ : Outport  Port=4  VectorParamsAs1DForOutWhenUnconnected=off
  __UniqueOutportName__5__ : Outport  Port=5  VectorParamsAs1DForOutWhenUnconnected=off
  __UniqueOutportName__6__ : Outport  Port=6  VectorParamsAs1DForOutWhenUnconnected=off
  __UniqueOutportName__7__ : Outport  Port=7  VectorParamsAs1DForOutWhenUnconnected=off
  wires:
  6DOF Bus/1 -> temporaryBusSelectName_1/1
  temporaryBusSelectName_1/1 -> __UniqueOutportName__1__/1  "<Ve>"
  temporaryBusSelectName_1/2 -> __UniqueOutportName__2__/1  "<Xe>"
  temporaryBusSelectName_1/3 -> __UniqueOutportName__3__/1  "<Eular(rad)>"
  temporaryBusSelectName_1/4 -> __UniqueOutportName__4__/1  "<DCM>"
  temporaryBusSelectName_1/5 -> __UniqueOutportName__5__/1  "<Vb>"
  temporaryBusSelectName_1/6 -> __UniqueOutportName__6__/1  "<wb>"
  temporaryBusSelectName_1/7 -> __UniqueOutportName__7__/1  "<dwb/dt>"

== system quadFly/Quadcopter Dynamics/Fail Model/__OutputSSForSFun__ ==
  __UniqueInportName__1__ : Inport
  __UniqueInportName__2__ : Inport  Port=2
  __UniqueInportName__3__ : Inport  Port=3
  Mux1 : BusCreator  Inputs=3
  Fail Model Bus : Outport  VectorParamsAs1DForOutWhenUnconnected=off
  wires:
  __UniqueInportName__1__/1 -> Mux1/1  "m"
  __UniqueInportName__2__/1 -> Mux1/2  "J"
  __UniqueInportName__3__/1 -> Mux1/3  "dM"
  Mux1/1 -> Fail Model Bus/1

== system quadFly/Quadcopter Dynamics/Force and Moment Model/__InputSSForSFun__ ==
  MotorRads : Inport
  Environment Model Bus : Inport  Port=2
  6DOF Bus : Inport  Port=3
  Fail Model Bus : Inport  Port=4
  "tZ " : Inport  Port=5
  temporaryBusSelectName_1 : BusSelector  OutputSignals=PosGPS,gravity,TempC,AirPressure,Rho,Windb,Wind
  temporaryBusSelectName_2 : BusSelector  OutputSignals=Ve,Xe,Eular(rad),DCM,Vb,wb,dwb/dt
  temporaryBusSelectName_3 : BusSelector  OutputSignals=m,J,dM
  __UniqueOutportName__1__ : Outport  VectorParamsAs1DForOutWhenUnconnected=off
  __UniqueOutportName__2__ : Outport  Port=2  VectorParamsAs1DForOutWhenUnconnected=off
  __UniqueOutportName__3__ : Outport  Port=3  VectorParamsAs1DForOutWhenUnconnected=off
  __UniqueOutportName__4__ : Outport  Port=4  VectorParamsAs1DForOutWhenUnconnected=off
  __UniqueOutportName__5__ : Outport  Port=5  VectorParamsAs1DForOutWhenUnconnected=off
  __UniqueOutportName__6__ : Outport  Port=6  VectorParamsAs1DForOutWhenUnconnected=off
  __UniqueOutportName__7__ : Outport  Port=7  VectorParamsAs1DForOutWhenUnconnected=off
  __UniqueOutportName__8__ : Outport  Port=8  VectorParamsAs1DForOutWhenUnconnected=off
  __UniqueOutportName__9__ : Outport  Port=9  VectorParamsAs1DForOutWhenUnconnected=off
  __UniqueOutportName__10__ : Outport  Port=10  VectorParamsAs1DForOutWhenUnconnected=off
  __UniqueOutportName__11__ : Outport  Port=11  VectorParamsAs1DForOutWhenUnconnected=off
  __UniqueOutportName__12__ : Outport  Port=12  VectorParamsAs1DForOutWhenUnconnected=off
  __UniqueOutportName__13__ : Outport  Port=13  VectorParamsAs1DForOutWhenUnconnected=off
  __UniqueOutportName__14__ : Outport  Port=14  VectorParamsAs1DForOutWhenUnconnected=off
  __UniqueOutportName__15__ : Outport  Port=15  VectorParamsAs1DForOutWhenUnconnected=off
  __UniqueOutportName__16__ : Outport  Port=16  VectorParamsAs1DForOutWhenUnconnected=off
  __UniqueOutportName__17__ : Outport  Port=17  VectorParamsAs1DForOutWhenUnconnected=off
  __UniqueOutportName__18__ : Outport  Port=18  VectorParamsAs1DForOutWhenUnconnected=off
  __UniqueOutportName__19__ : Outport  Port=19  VectorParamsAs1DForOutWhenUnconnected=off
  wires:
  Environment Model Bus/1 -> temporaryBusSelectName_1/1
  6DOF Bus/1 -> temporaryBusSelectName_2/1
  Fail Model Bus/1 -> temporaryBusSelectName_3/1
  MotorRads/1 -> __UniqueOutportName__1__/1
  temporaryBusSelectName_1/1 -> __UniqueOutportName__2__/1  "<PosGPS>"
  temporaryBusSelectName_1/2 -> __UniqueOutportName__3__/1  "<gravity>"
  temporaryBusSelectName_1/3 -> __UniqueOutportName__4__/1  "<TempC>"
  temporaryBusSelectName_1/4 -> __UniqueOutportName__5__/1  "<AirPressure>"
  temporaryBusSelectName_1/5 -> __UniqueOutportName__6__/1  "<Rho>"
  temporaryBusSelectName_1/6 -> __UniqueOutportName__7__/1  "<Windb>"
  temporaryBusSelectName_1/7 -> __UniqueOutportName__8__/1  "<Wind>"
  temporaryBusSelectName_2/1 -> __UniqueOutportName__9__/1  "<Ve>"
  temporaryBusSelectName_2/2 -> __UniqueOutportName__10__/1  "<Xe>"
  temporaryBusSelectName_2/3 -> __UniqueOutportName__11__/1  "<Eular(rad)>"
  temporaryBusSelectName_2/4 -> __UniqueOutportName__12__/1  "<DCM>"
  temporaryBusSelectName_2/5 -> __UniqueOutportName__13__/1  "<Vb>"
  temporaryBusSelectName_2/6 -> __UniqueOutportName__14__/1  "<wb>"
  temporaryBusSelectName_2/7 -> __UniqueOutportName__15__/1  "<dwb/dt>"
  temporaryBusSelectName_3/1 -> __UniqueOutportName__16__/1  "<m>"
  temporaryBusSelectName_3/2 -> __UniqueOutportName__17__/1  "<J>"
  temporaryBusSelectName_3/3 -> __UniqueOutportName__18__/1  "<dM>"
  "tZ "/1 -> __UniqueOutportName__19__/1

== system quadFly/Quadcopter Dynamics/Force and Moment Model/__OutputSSForSFun__ ==
  __UniqueInportName__1__ : Inport
  __UniqueInportName__2__ : Inport  Port=2
  __UniqueInportName__3__ : Inport  Port=3
  Mux1 : BusCreator  Inputs=3
  Force and Moment Model Bus : Outport  VectorParamsAs1DForOutWhenUnconnected=off
  wires:
  __UniqueInportName__1__/1 -> Mux1/1  "Fb"
  __UniqueInportName__2__/1 -> Mux1/2  "Mb"
  __UniqueInportName__3__/1 -> Mux1/3  "landed"
  Mux1/1 -> Force and Moment Model Bus/1

== system quadFly/Quadcopter Dynamics/Motor Model/__InputSSForSFun__ ==
  Battery Model Bus : Inport
  temporaryBusSelectName_1 : BusSelector  OutputSignals=PWMOut,cellVol,remCapa
  __UniqueOutportName__1__ : Outport  VectorParamsAs1DForOutWhenUnconnected=off
  __UniqueOutportName__2__ : Outport  Port=2  VectorParamsAs1DForOutWhenUnconnected=off
  __UniqueOutportName__3__ : Outport  Port=3  VectorParamsAs1DForOutWhenUnconnected=off
  wires:
  Battery Model Bus/1 -> temporaryBusSelectName_1/1
  temporaryBusSelectName_1/1 -> __UniqueOutportName__1__/1  "<PWMOut>"
  temporaryBusSelectName_1/2 -> __UniqueOutportName__2__/1  "<cellVol>"
  temporaryBusSelectName_1/3 -> __UniqueOutportName__3__/1  "<remCapa>"

== system quadFly/Quadcopter Dynamics/Motor Model/__OutputSSForSFun__ ==
  __UniqueInportName__1__ : Inport
  MotorRads : Outport  VectorParamsAs1DForOutWhenUnconnected=off
  wires:
  __UniqueInportName__1__/1 -> MotorRads/1  "y"

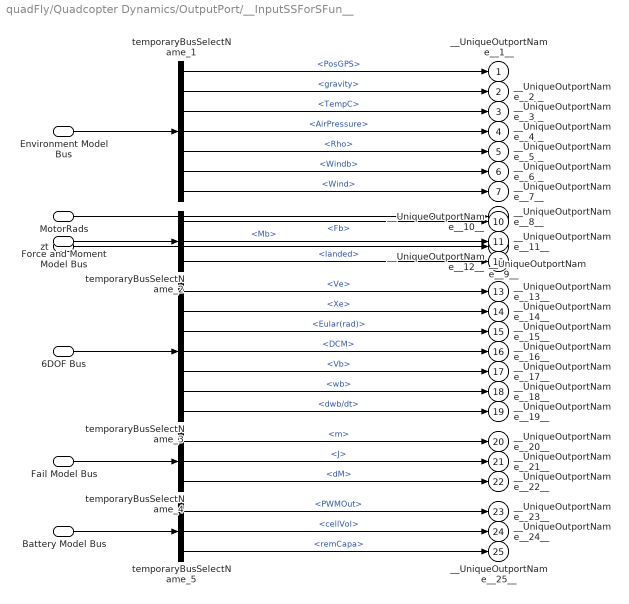
== system quadFly/Quadcopter Dynamics/OutputPort/__InputSSForSFun__ ==
  Environment Model Bus : Inport
  MotorRads : Inport  Port=2
  zt : Inport  Port=3
  Force and Moment Model Bus : Inport  Port=4
  6DOF Bus : Inport  Port=5
  Fail Model Bus : Inport  Port=6
  Battery Model Bus : Inport  Port=7
  temporaryBusSelectName_1 : BusSelector  OutputSignals=PosGPS,gravity,TempC,AirPressure,Rho,Windb,Wind
  temporaryBusSelectName_2 : BusSelector  OutputSignals=Fb,Mb,landed
  temporaryBusSelectName_3 : BusSelector  OutputSignals=Ve,Xe,Eular(rad),DCM,Vb,wb,dwb/dt
  temporaryBusSelectName_4 : BusSelector  OutputSignals=m,J,dM
  temporaryBusSelectName_5 : BusSelector  OutputSignals=PWMOut,cellVol,remCapa
  __UniqueOutportName__1__ : Outport  VectorParamsAs1DForOutWhenUnconnected=off
  __UniqueOutportName__2__ : Outport  Port=2  VectorParamsAs1DForOutWhenUnconnected=off
  __UniqueOutportName__3__ : Outport  Port=3  VectorParamsAs1DForOutWhenUnconnected=off
  __UniqueOutportName__4__ : Outport  Port=4  VectorParamsAs1DForOutWhenUnconnected=off
  __UniqueOutportName__5__ : Outport  Port=5  VectorParamsAs1DForOutWhenUnconnected=off
  __UniqueOutportName__6__ : Outport  Port=6  VectorParamsAs1DForOutWhenUnconnected=off
  __UniqueOutportName__7__ : Outport  Port=7  VectorParamsAs1DForOutWhenUnconnected=off
  __UniqueOutportName__8__ : Outport  Port=8  VectorParamsAs1DForOutWhenUnconnected=off
  __UniqueOutportName__9__ : Outport  Port=9  VectorParamsAs1DForOutWhenUnconnected=off
  __UniqueOutportName__10__ : Outport  Port=10  VectorParamsAs1DForOutWhenUnconnected=off
  __UniqueOutportName__11__ : Outport  Port=11  VectorParamsAs1DForOutWhenUnconnected=off
  __UniqueOutportName__12__ : Outport  Port=12  VectorParamsAs1DForOutWhenUnconnected=off
  __UniqueOutportName__13__ : Outport  Port=13  VectorParamsAs1DForOutWhenUnconnected=off
  __UniqueOutportName__14__ : Outport  Port=14  VectorParamsAs1DForOutWhenUnconnected=off
  __UniqueOutportName__15__ : Outport  Port=15  VectorParamsAs1DForOutWhenUnconnected=off
  __UniqueOutportName__16__ : Outport  Port=16  VectorParamsAs1DForOutWhenUnconnected=off
  __UniqueOutportName__17__ : Outport  Port=17  VectorParamsAs1DForOutWhenUnconnected=off
  __UniqueOutportName__18__ : Outport  Port=18  VectorParamsAs1DForOutWhenUnconnected=off
  __UniqueOutportName__19__ : Outport  Port=19  VectorParamsAs1DForOutWhenUnconnected=off
  __UniqueOutportName__20__ : Outport  Port=20  VectorParamsAs1DForOutWhenUnconnected=off
  __UniqueOutportName__21__ : Outport  Port=21  VectorParamsAs1DForOutWhenUnconnected=off
  __UniqueOutportName__22__ : Outport  Port=22  VectorParamsAs1DForOutWhenUnconnected=off
  __UniqueOutportName__23__ : Outport  Port=23  VectorParamsAs1DForOutWhenUnconnected=off
  __UniqueOutportName__24__ : Outport  Port=24  VectorParamsAs1DForOutWhenUnconnected=off
  __UniqueOutportName__25__ : Outport  Port=25  VectorParamsAs1DForOutWhenUnconnected=off
  wires:
  Environment Model Bus/1 -> temporaryBusSelectName_1/1
  Force and Moment Model Bus/1 -> temporaryBusSelectName_2/1
  6DOF Bus/1 -> temporaryBusSelectName_3/1
  Fail Model Bus/1 -> temporaryBusSelectName_4/1
  Battery Model Bus/1 -> temporaryBusSelectName_5/1
  temporaryBusSelectName_1/1 -> __UniqueOutportName__1__/1  "<PosGPS>"
  temporaryBusSelectName_1/2 -> __UniqueOutportName__2__/1  "<gravity>"
  temporaryBusSelectName_1/3 -> __UniqueOutportName__3__/1  "<TempC>"
  temporaryBusSelectName_1/4 -> __UniqueOutportName__4__/1  "<AirPressure>"
  temporaryBusSelectName_1/5 -> __UniqueOutportName__5__/1  "<Rho>"
  temporaryBusSelectName_1/6 -> __UniqueOutportName__6__/1  "<Windb>"
  temporaryBusSelectName_1/7 -> __UniqueOutportName__7__/1  "<Wind>"
  MotorRads/1 -> __UniqueOutportName__8__/1
  zt/1 -> __UniqueOutportName__9__/1
  temporaryBusSelectName_2/1 -> __UniqueOutportName__10__/1  "<Fb>"
  temporaryBusSelectName_2/2 -> __UniqueOutportName__11__/1  "<Mb>"
  temporaryBusSelectName_2/3 -> __UniqueOutportName__12__/1  "<landed>"
  temporaryBusSelectName_3/1 -> __UniqueOutportName__13__/1  "<Ve>"
  temporaryBusSelectName_3/2 -> __UniqueOutportName__14__/1  "<Xe>"
  temporaryBusSelectName_3/3 -> __UniqueOutportName__15__/1  "<Eular(rad)>"
  temporaryBusSelectName_3/4 -> __UniqueOutportName__16__/1  "<DCM>"
  temporaryBusSelectName_3/5 -> __UniqueOutportName__17__/1  "<Vb>"
  temporaryBusSelectName_3/6 -> __UniqueOutportName__18__/1  "<wb>"
  temporaryBusSelectName_3/7 -> __UniqueOutportName__19__/1  "<dwb/dt>"
  temporaryBusSelectName_4/1 -> __UniqueOutportName__20__/1  "<m>"
  temporaryBusSelectName_4/2 -> __UniqueOutportName__21__/1  "<J>"
  temporaryBusSelectName_4/3 -> __UniqueOutportName__22__/1  "<dM>"
  temporaryBusSelectName_5/1 -> __UniqueOutportName__23__/1  "<PWMOut>"
  temporaryBusSelectName_5/2 -> __UniqueOutportName__24__/1  "<cellVol>"
  temporaryBusSelectName_5/3 -> __UniqueOutportName__25__/1  "<remCapa>"

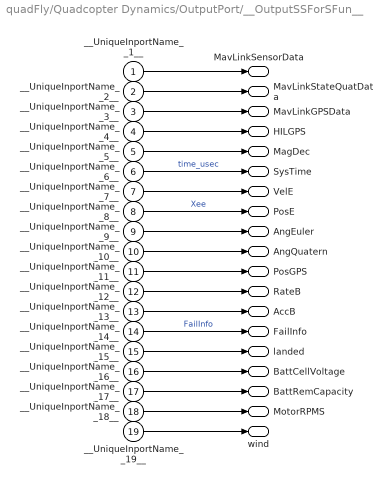
== system quadFly/Quadcopter Dynamics/OutputPort/__OutputSSForSFun__ ==
  __UniqueInportName__1__ : Inport
  __UniqueInportName__2__ : Inport  Port=2
  __UniqueInportName__3__ : Inport  Port=3
  __UniqueInportName__4__ : Inport  Port=4
  __UniqueInportName__5__ : Inport  Port=5
  __UniqueInportName__6__ : Inport  Port=6
  __UniqueInportName__7__ : Inport  Port=7
  __UniqueInportName__8__ : Inport  Port=8
  __UniqueInportName__9__ : Inport  Port=9
  __UniqueInportName__10__ : Inport  Port=10
  __UniqueInportName__11__ : Inport  Port=11
  __UniqueInportName__12__ : Inport  Port=12
  __UniqueInportName__13__ : Inport  Port=13
  __UniqueInportName__14__ : Inport  Port=14
  __UniqueInportName__15__ : Inport  Port=15
  __UniqueInportName__16__ : Inport  Port=16
  __UniqueInportName__17__ : Inport  Port=17
  __UniqueInportName__18__ : Inport  Port=18
  __UniqueInportName__19__ : Inport  Port=19
  MavLinkSensorData : Outport  OutDataTypeStr=Bus: MavLinkSensor  SampleTime=[-1 0]  VectorParamsAs1DForOutWhenUnconnected=off  BusOutputAsStruct=on
  MavLinkStateQuatData : Outport  Port=2  OutDataTypeStr=Bus: MavLinkStateQuat  SampleTime=[-1 0]  VectorParamsAs1DForOutWhenUnconnected=off  BusOutputAsStruct=on
  MavLinkGPSData : Outport  Port=3  OutDataTypeStr=Bus: MavLinkGPS  SampleTime=[-1 0]  VectorParamsAs1DForOutWhenUnconnected=off  BusOutputAsStruct=on
  HILGPS : Outport  Port=4  OutDataTypeStr=Bus: HILGPS  SampleTime=[-1 0]  VectorParamsAs1DForOutWhenUnconnected=off  BusOutputAsStruct=on
  MagDec : Outport  Port=5  VectorParamsAs1DForOutWhenUnconnected=off
  SysTime : Outport  Port=6  VectorParamsAs1DForOutWhenUnconnected=off
  VelE : Outport  Port=7  VectorParamsAs1DForOutWhenUnconnected=off
  PosE : Outport  Port=8  VectorParamsAs1DForOutWhenUnconnected=off
  AngEuler : Outport  Port=9  VectorParamsAs1DForOutWhenUnconnected=off
  AngQuatern : Outport  Port=10  VectorParamsAs1DForOutWhenUnconnected=off
  PosGPS : Outport  Port=11  VectorParamsAs1DForOutWhenUnconnected=off
  RateB : Outport  Port=12  VectorParamsAs1DForOutWhenUnconnected=off
  AccB : Outport  Port=13  VectorParamsAs1DForOutWhenUnconnected=off
  FailInfo : Outport  Port=14  VectorParamsAs1DForOutWhenUnconnected=off
  landed : Outport  Port=15  VectorParamsAs1DForOutWhenUnconnected=off
  BattCellVoltage : Outport  Port=16  VectorParamsAs1DForOutWhenUnconnected=off
  BattRemCapacity : Outport  Port=17  VectorParamsAs1DForOutWhenUnconnected=off
  MotorRPMS : Outport  Port=18  VectorParamsAs1DForOutWhenUnconnected=off
  wind : Outport  Port=19  VectorParamsAs1DForOutWhenUnconnected=off
  wires:
  __UniqueInportName__1__/1 -> MavLinkSensorData/1
  __UniqueInportName__2__/1 -> MavLinkStateQuatData/1
  __UniqueInportName__3__/1 -> MavLinkGPSData/1
  __UniqueInportName__4__/1 -> HILGPS/1
  __UniqueInportName__5__/1 -> MagDec/1
  __UniqueInportName__6__/1 -> SysTime/1  "time_usec"
  __UniqueInportName__7__/1 -> VelE/1
  __UniqueInportName__8__/1 -> PosE/1  "Xee"
  __UniqueInportName__9__/1 -> AngEuler/1
  __UniqueInportName__10__/1 -> AngQuatern/1
  __UniqueInportName__11__/1 -> PosGPS/1
  __UniqueInportName__12__/1 -> RateB/1
  __UniqueInportName__13__/1 -> AccB/1
  __UniqueInportName__14__/1 -> FailInfo/1  "FailInfo"
  __UniqueInportName__15__/1 -> landed/1
  __UniqueInportName__16__/1 -> BattCellVoltage/1
  __UniqueInportName__17__/1 -> BattRemCapacity/1
  __UniqueInportName__18__/1 -> MotorRPMS/1
  __UniqueInportName__19__/1 -> wind/1
